simulink model "verify_Pipe_Geometry_mdl"  (R2016b)
settings: Solver=ode45  StartTime=0.0  StopTime=150  MaxStep=5  RelTol=1e-3  EnableMultiTasking=on
libraries: carnot x3
settings Model: Creator=drhf  LastModifiedBy=drhf
settings DataIOCC: SaveFormat=Array  SignalLoggingSaveFormat=ModelDataLogs
settings OptimizationCC: ExpressionDepthLimit=2147483647  LifeSpan=inf
settings DebuggingCC: UnderspecifiedInitializationDetection=Classic  MergeDetectMultiDrivingBlocksExec=none  SolverPrmCheckMsg=warning  FcnCallInpInsideContextMsg=warning  StateNameClashWarn=warning  SFUnexpectedBacktrackingDiag=warning  SFNoUnconditionalDefaultTransitionDiag=warning  SFExecutionAtInitializationDiag=none
settings HardwareCC: ProdBitPerPointer=32  ProdBitPerSizeT=32  ProdBitPerPtrDiffT=32  ProdLargestAtomicFloat=None  ProdIntDivRoundTo=Undefined  ProdEndianess=Unspecified  ProdWordSize=32  ProdHWDeviceType=32-bit Generic
settings ModelReferenceCC: PropagateSignalLabelsOutOfModel=off
settings GRTTargetCC: TargetLangStandard=C89/C90 (ANSI)  GeneratePreprocessorConditionals=Disable all  CombineOutputUpdateFcns=off  GRTInterface=on
settings ConfigComp: CovMetricSettings=dw  CovHtmlReporting=on  CovSaveCumulativeToWorkspaceVar=on  CovSaveSingleToWorkspaceVar=on  CovExternalEMLEnable=off

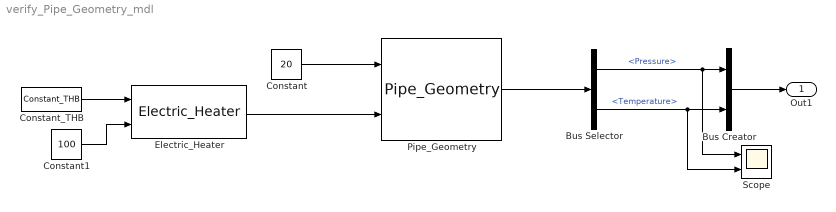
== system verify_Pipe_Geometry_mdl ==
  Bus Creator : BusCreator  Inputs=2
  Bus Selector : BusSelector  OutputSignals=Pressure,Temperature
  Constant : Constant  Value=20
  Constant1 : Constant  Value=100
  Constant_THB : carnot/Source/Simple/Constant_THB  t=40  mdot=720/3600  p=2e5  mID=Full Pressure Drop with Static Height  fluid=Water  mix=0  mix2=0  mix3=0  dia=10  hgt=0
  Electric_Heater : carnot/Source/Boiler/Electric_Heater
  Pipe_Geometry : carnot/Hydraulics/Pipe_Geometry  dia=0.02  len=10  hgt=10  uloss=100/20/10  cond=0  cwall=1000  t0=20  rough=0.04*1e-3  nbend=4  nodes=1
  Scope : Scope  NumInputPorts=2
  Out1 : Outport
  wires:
  Bus Creator/1 -> Out1/1
  Bus Selector/1 -> Scope/1, Bus Creator/1  "<Pressure>"
  Bus Selector/2 -> Scope/2, Bus Creator/2  "<Temperature>"
  Constant_THB/1 -> Electric_Heater/1
  Constant/1 -> Pipe_Geometry/1
  Electric_Heater/1 -> Pipe_Geometry/2
  Pipe_Geometry/1 -> Bus Selector/1
  Constant1/1 -> Electric_Heater/2
